simulink model "Correction"  (R2021b)
settings: Solver=VariableStepAuto  StartTime=0.0  StopTime=10.0  RelTol=1e-3
libraries: simulink x2
settings Model: Creator=ygx  LastModifiedBy=ygx

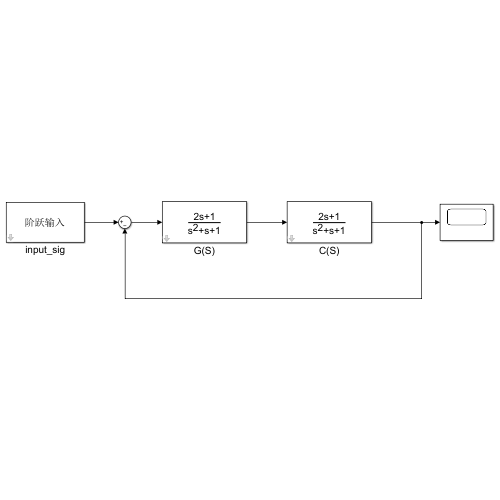
[thumbnail: Simulink's stored preview of the top-level diagram]
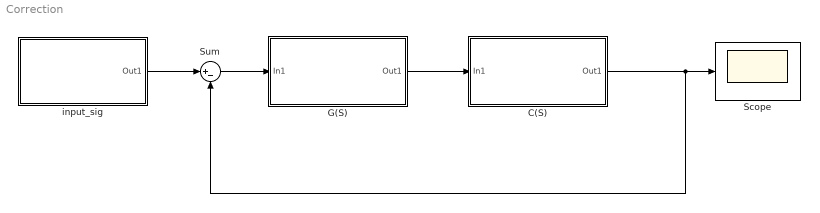
== system Correction ==
  C(S) : Subsystem  mask{K1=[0 2 1], den_g=[1 1 1]}
      mask prompts: K1 "K"; den_g "参数输入"
      mask DialogControl DescGroupVar Prompt: G(s)分子参数设置
      mask DialogControl ParameterGroupVar Prompt: G(S)分母参数设置
      mask Display: dpoly([0 0 K1],den_g, 's')
  G(S) : Subsystem  mask{K1=[0 2 1], den_g=[1 1 1]}
      mask prompts: K1 "K"; den_g "参数输入"
      mask DialogControl DescGroupVar Prompt: G(s)分子参数设置
      mask DialogControl ParameterGroupVar Prompt: G(S)分母参数设置
      mask Display: dpoly([0 0 K1],den_g, 's')
  Scope : Scope
  Sum : Sum  Inputs=|+-
  input_sig : Subsystem  mask{input_num=阶跃信号, step_time=0, step_init=0, step_final=1}
      mask prompts: input_num "信号输入选择"; step_time "阶跃时间"; step_init "初值"; step_final "终值"
      mask TypeOptions input_num: 阶跃信号 | 斜坡信号 | 加速度信号 | 正弦信号
      mask DialogControl Control1 Prompt: 阶跃信号参数设置
      mask Display:
      | if input_num==1
      |     disp('阶跃输入');
      | elseif input_num==2
      |     disp('斜坡（速度）输入');
      | elseif input_num==3
      |     disp('加速度输入');
      | elseif input_num==4
      |     disp('正弦');
      | else
      |     disp('输入信号选择');
      | end
  wires:
  Sum/1 -> G(S)/1(In1)
  input_sig/1(Out1) -> Sum/1
  G(S)/1(Out1) -> C(S)/1(In1)
  C(S)/1(Out1) -> Sum/2, Scope/1

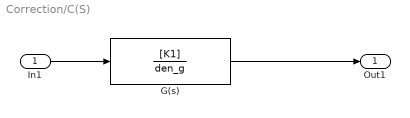
== system Correction/C(S) ==
  In1 : Inport
  G(s) : TransferFcn  Numerator=[K1]  Denominator=den_g  ContinuousStateAttributes='position'
  Out1 : Outport
  wires:
  G(s)/1 -> Out1/1
  In1/1 -> G(s)/1

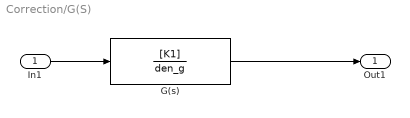
== system Correction/G(S) ==
  In1 : Inport
  G(s) : TransferFcn  Numerator=[K1]  Denominator=den_g  ContinuousStateAttributes='position'
  Out1 : Outport
  wires:
  G(s)/1 -> Out1/1
  In1/1 -> G(s)/1

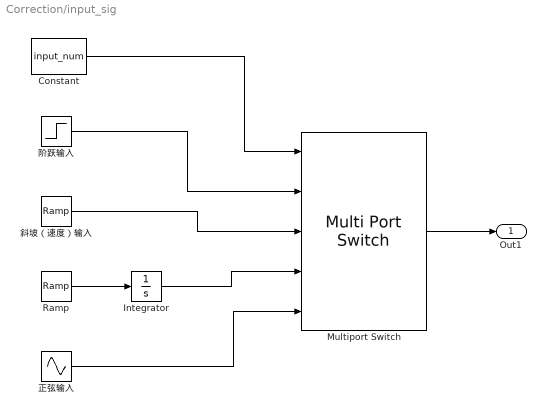
== system Correction/input_sig ==
  Constant : Constant  Value=input_num
  Integrator : Integrator
  Multiport Switch : MultiPortSwitch  Inputs=4
  Ramp : simulink/Sources/Ramp  slope=1  start=0  InitialOutput=0
  斜坡（速度）输入 : simulink/Sources/Ramp  slope=1  start=0  InitialOutput=0
  正弦输入 : Sin  SampleTime=0
  阶跃输入 : Step  Time=step_time  Before=step_init  After=step_final  SampleTime=0
  Out1 : Outport
  wires:
  Ramp/1 -> Integrator/1
  阶跃输入/1 -> Multiport Switch/2
  斜坡（速度）输入/1 -> Multiport Switch/3
  Integrator/1 -> Multiport Switch/4
  Multiport Switch/1 -> Out1/1
  正弦输入/1 -> Multiport Switch/5
  Constant/1 -> Multiport Switch/1
